simulink model "MBSE_PROJECT"  (R2020b)
settings: Solver=VariableStepAuto  StartTime=0.0  StopTime=10.0  RelTol=1e-3
undefined symbols (not defined in the file): sigbuilder_block
libraries: simulink x18
(part 1 of 2)
settings Model: Creator=99003757  LastModifiedBy=99003732

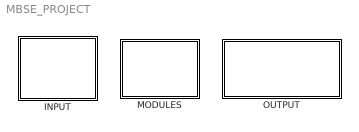
== system MBSE_PROJECT ==
  INPUT : Subsystem
  MODULES : Subsystem
  OUTPUT : Subsystem

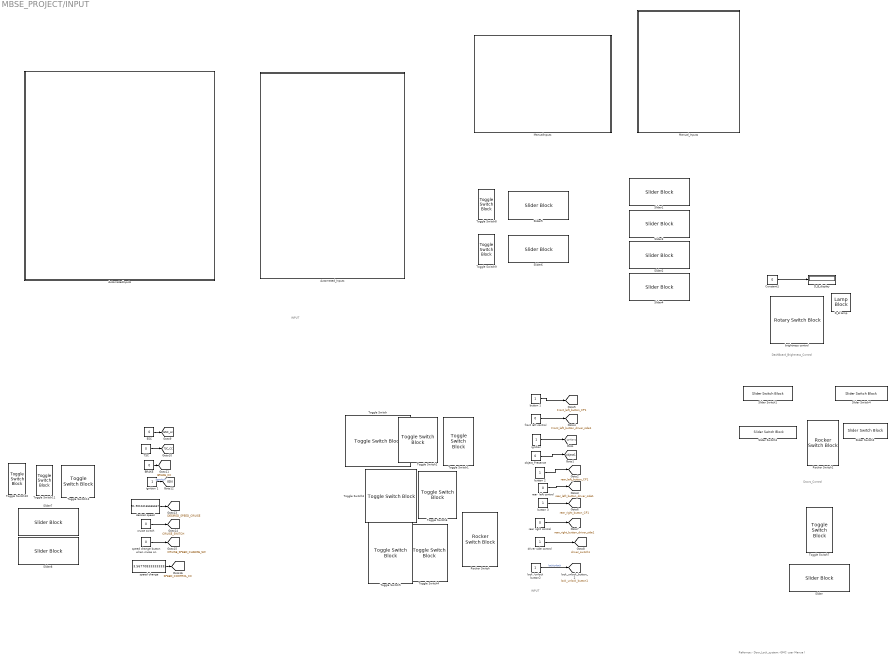
== system MBSE_PROJECT/INPUT ==
  note: INPUT
  note: INPUT
  note: DashBoard_Brightness_Control
  note: Doors_Control
  note: Refernce:-
      | Door_Lock_system:-GMC user Manua l
  AutomatedInputs : Subsystem
  Automated_Inputs : Subsystem
  BRAKE : Constant  Value=0
  Constant1 : Constant  Value=0
  D_B lamp : LampBlock
  D_B_display : Display
  ESC : Constant  Value=0
  ManualInputs : Subsystem
  Manual_Inputs : Subsystem
  Rocker Switch : RockerSwitchBlock  LabelPosition=Bottom
      settings: Values={{'Off', 'On'}, [0 1]}
  Rocker Switch1 : RockerSwitchBlock
      settings: Values={{'Off', 'On'}, [1 0]}
  Slider{,1..8} (9 alike) : SliderBlock
  Slider Switch{1..4} (4 alike) : SliderSwitchBlock
      settings: Values={{'unlock', 'lock'}, [0 1]}
  TSC : Constant  Value=0
  Toggle Switch{,1..12} (13 alike) : ToggleSwitchBlock
  brightness control : RotarySwitchBlock
      settings: Values={{'Off', 'very Low', 'Low', 'medium', 'high', 'very high'}, [0 1 2 3 4 5]}
  "button 1 " : Constant
  button 2 : Constant
  button 3 : Constant
  cruise switch : Constant  Value=0
  desired speed : Constant  Value=51.90104166666667
  driver side control : Constant
  front left control : Constant  Value=0
  "ignition " : Constant
  ignition 1 : Constant
  lock /unlock button2 : Constant
  object_Presence : Constant  Value=0
  rear  left control : Constant  Value=0
  rear right control : Constant  Value=0
  speed change : Constant  Value=3.567708333333333
  "speed change button when cruise on " : Constant  Value=0
  tag scope: BRAKE_CC=global, CRUISE_SPEED_CHANGE_SW=global, CRUISE_SWITCH=global, DESIRED_SPEED_CRUISE=global, ESC_cc=global, Front_left_button_CP1=global, Front_left_button_driver_side1=global, IGN=global, SPEED_CONTROL_CC=global, TSC_CC=global, driver_switch1=global, ignition1=global, lock_unlock_button1=global, object1=global, rear_left_button_CP1=global, rear_left_button_driver_side1=global, rear_right_button_CP1=global, rear_right_button_driver_side1=global
  wires:
  object_Presence/1 -> [object1]
  driver side control/1 -> [driver_switch1]
  Constant1/1 -> D_B_display/1
  button 3/1 -> [rear_right_button_CP1]
  rear right control/1 -> [rear_right_button_driver_side1]
  "ignition "/1 -> [ignition1]
  rear  left control/1 -> [rear_left_button_driver_side1]
  lock /unlock button2/1 -> [lock_unlock_button1]  "lock/unlock"
  button 2/1 -> [rear_left_button_CP1]
  front left control/1 -> [Front_left_button_driver_side1]
  "button 1 "/1 -> [Front_left_button_CP1]
  speed change/1 -> [SPEED_CONTROL_CC]
  desired speed/1 -> [DESIRED_SPEED_CRUISE]
  ESC/1 -> [ESC_cc]
  ignition 1/1 -> [IGN]  "igswitch"
  "speed change button when cruise on "/1 -> [CRUISE_SPEED_CHANGE_SW]
  BRAKE/1 -> [BRAKE_CC]
  TSC/1 -> [TSC_CC]
  cruise switch/1 -> [CRUISE_SWITCH]

== system MBSE_PROJECT/MODULES ==
  "\tPOWER_WINDOW" : Subsystem
  AirBagSystem : Subsystem
  CRUISE_CONTROL : Subsystem
  SeatRestraintSystem : Subsystem
  Subsystem2 : Subsystem
  Subsystem4 : Subsystem
  Tire Pressure Monitoring System : Subsystem

== system MBSE_PROJECT/OUTPUT ==
  note: Roof light
  note: Signal status
  note: roof light
  Cruise_output : Subsystem
  Lamp : LampBlock
  OUTPUT : Subsystem
  OUTPUT1 : Subsystem
  Outputs : Subsystem
  Outputs_Display : Subsystem
  TP1_Indicator : LampBlock
  TP2_Indicator : LampBlock
  TP3_Indicator : LampBlock
  TP4_Indicator : LampBlock
  automatic door lamp status : LampBlock
  delay lamp status : LampBlock

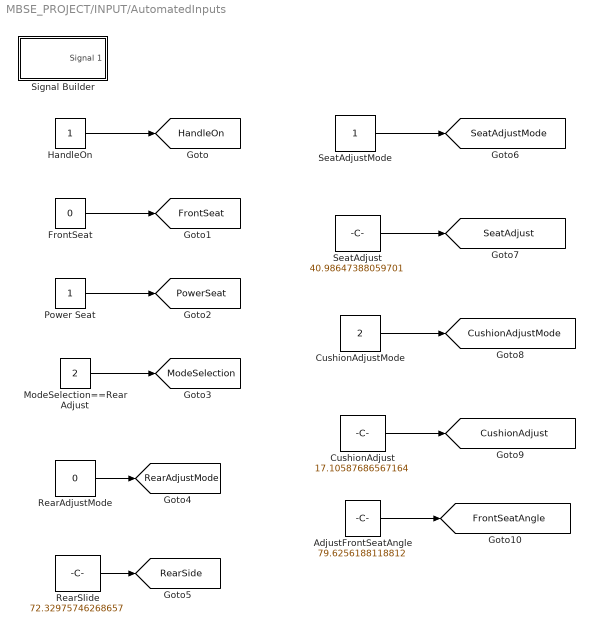
== system MBSE_PROJECT/INPUT/AutomatedInputs ==
  AdjustFrontSeatAngle : Constant  Value=79.6256188118812
  CushionAdjust : Constant  Value=17.10587686567164
  CushionAdjustMode : Constant  Value=2
  FrontSeat : Constant  Value=0
  HandleOn : Constant
  ModeSelection==RearAdjust : Constant  Value=2
  Power Seat : Constant
  RearAdjustMode : Constant  Value=0
  RearSlide : Constant  Value=72.32975746268657
  SeatAdjust : Constant  Value=40.98647388059701
  SeatAdjustMode : Constant
  Signal Builder : Subsystem  Tag=STV Subsys  LoadFcn=sigbuilder_block('load');  StartFcn=sigbuilder_block('start');  StopFcn=sigbuilder_block('stop');  ClipboardFcn=sigbuilder_block('clipboard');  mask(Sigbuilder block){tuvar=[0:10]}
      mask help: Simulink:masks:SigbuilderBlock_MD
      mask init:
      | if ~strcmp(get_param(bdroot(gcbh),'SimulationStatus'),'stopped') tuvar = sigbuilder_block('maskInit'); end
      settings: CopyFcn=sigbuilder_block('copy');  DeleteFcn=sigbuilder_block('delete');  ModelCloseFcn=sigbuilder_block('modelClose');  PreSaveFcn=sigbuilder_block('preSave');  PauseFcn=sigbuilder_block('pause');  ContinueFcn=sigbuilder_block('continue');  NameChangeFcn=sigbuilder_block('namechange');  OpenFcn=sigbuilder_block('open',[437.6 199.2 550.4 400 ]);  CloseFcn=sigbuilder_block('close');
      mask Display: plot(0, 0, 100, 100,[2, 2, 32, 32, 2], [68, 8, 8, 68, 68],[32, 2], [38, 38], [32, 19, 2],[53, 60, 44], [32, 17, 17, 2],[16, 16, 31, 31]);txt = getActiveGroup(gcbh);text(2, 100, txt,'verticalAlignment', 'top');
  tag scope: CushionAdjust=global, CushionAdjustMode=global, FrontSeat=global, FrontSeatAngle=global, HandleOn=global, ModeSelection=global, PowerSeat=global, RearAdjustMode=global, RearSide=global, SeatAdjust=global, SeatAdjustMode=global
  wires:
  HandleOn/1 -> [HandleOn]
  FrontSeat/1 -> [FrontSeat]
  Power Seat/1 -> [PowerSeat]
  ModeSelection==RearAdjust/1 -> [ModeSelection]
  RearAdjustMode/1 -> [RearAdjustMode]
  RearSlide/1 -> [RearSide]
  SeatAdjustMode/1 -> [SeatAdjustMode]
  SeatAdjust/1 -> [SeatAdjust]
  CushionAdjustMode/1 -> [CushionAdjustMode]
  CushionAdjust/1 -> [CushionAdjust]
  AdjustFrontSeatAngle/1 -> [FrontSeatAngle]

== system MBSE_PROJECT/INPUT/Automated_Inputs ==
  Driver : Constant
  L_Front : Constant
  L_Rear : Constant
  R_Rear : Constant  Value=0
  VehicleSpeed : Constant  Value=180
  YawRate : Constant  Value=100
  tag scope: Driver=global, L_Front=global, L_Rear=global, R_Rear=global, VehicleSpeed=global, YawRate=global
  wires:
  VehicleSpeed/1 -> [VehicleSpeed]
  YawRate/1 -> [YawRate]
  Driver/1 -> [Driver]
  L_Front/1 -> [L_Front]
  L_Rear/1 -> [L_Rear]
  R_Rear/1 -> [R_Rear]

== system MBSE_PROJECT/INPUT/ManualInputs ==
  Rotary Switch : RotarySwitchBlock  Commented=on
      settings: Values={{'RearAdjust', 'SeatAdjust', 'CushionAdjust', 'Lock'}, [0 1 2 3]}
  Slider to set the position of Frontseat : SliderBlock  Commented=on
  SliderForCushionAdjust : SliderBlock  Commented=on
  SliderForRearAdjust : SliderBlock  Commented=on
  SliderForSeatAdjust1 : SliderBlock  Commented=on
  Toggle Switch1 : ToggleSwitchBlock  Commented=on
      settings: Values={{'Off', 'On'}, [0 1]}
  Toggle Switch2 : ToggleSwitchBlock  Commented=on
      settings: Values={{'Off', 'On'}, [0 1]}
  Toggle Switch3 : ToggleSwitchBlock  Commented=on
      settings: Values={{'Off', 'On'}, [0 1]}

== system MBSE_PROJECT/INPUT/Manual_Inputs ==
  Vehicle_Speed : RotarySwitchBlock  Commented=on
      settings: Values={{'50kmph', '80kmph', '100kmph', '140kmph', '180kmph', '230kmph'}, [50 80 100 140 180 230]}
  YawRateMeasure : RotarySwitchBlock  Commented=on
      settings: Values={{'Forward', 'Turning'}, [50 100]}

== system MBSE_PROJECT/MODULES/	POWER_WINDOW ==
  Subsystem4 : Subsystem
  tag scope: FL_out=global, FL_warn=global, RL_out=global, RL_warn=global, RR_out=global, RR_warn=global, driver_side_output=global, driver_warn=global
  wires:
  Subsystem4/2(Out_FL) -> [FL_out]
  Subsystem4/1(Out_warn) -> [FL_warn]
  Subsystem4/4(Out_RL) -> [RL_out]
  Subsystem4/6(Out_RR) -> [RR_out]
  [object1] -> Subsystem4/2(object)
  [ignition1] -> Subsystem4/1(Ig_sw)
  Subsystem4/3(Out_RL_warn) -> [RL_warn]
  Subsystem4/8(Out_DC) -> [driver_side_output]
  Subsystem4/5(Out_RR_warn) -> [RR_warn]
  Subsystem4/7(Out_DC_warn) -> [driver_warn]

== system MBSE_PROJECT/MODULES/AirBagSystem ==
  AND : Logic  IconShape=distinctive  AllPortsSameDT=off  OutDataTypeStr=boolean
  AND1 : Logic  IconShape=distinctive  AllPortsSameDT=off  OutDataTypeStr=boolean
  ActivateAirBagSensor : MATLAB Function  TreatAsAtomicUnit=on
  DetectDeceleration : Subsystem
  FrontAirBagActivation : Subsystem  TreatAsAtomicUnit=on
  Side/Front : Subsystem
  SideAirBagActivation : Subsystem  TreatAsAtomicUnit=on
  wires:
  AND/1 -> FrontAirBagActivation/1(True), FrontAirBagActivation/Enable
  Side/Front/2(In_Front1) -> AND1/1
  ActivateAirBagSensor/1(AirBagSensor) -> AND1/2, AND/2
  Side/Front/1(In_Front) -> AND/1
  AND1/1 -> SideAirBagActivation/1(True), SideAirBagActivation/Enable
  DetectDeceleration/1(Out1) -> ActivateAirBagSensor/1(SuddenDeceleration)

== system MBSE_PROJECT/MODULES/CRUISE_CONTROL ==
  note: IGN
  Display : Display
  MATLAB Function : MATLAB Function  TreatAsAtomicUnit=on
  tag scope: output_cruise=global
  wires:
  [DESIRED_SPEED_CRUISE] -> MATLAB Function/5(DESIRED_SPEED_CRUISE)
  [BRAKE_CC] -> MATLAB Function/3(BRAKE_CC)
  [CRUISE_SWITCH] -> MATLAB Function/6(cs)
  [ESC_cc] -> MATLAB Function/1(ESC_CC)
  [SPEED_CONTROL_CC] -> MATLAB Function/8(speedch)
  MATLAB Function/1(y) -> [output_cruise], Display/1  "output"
  [TSC_CC] -> MATLAB Function/2(TSC_CC)
  [IGN] -> MATLAB Function/4(IGN)
  [CRUISE_SPEED_CHANGE_SW] -> MATLAB Function/7(CRUISE_SPEED_CHANGE_SW)

== system MBSE_PROJECT/MODULES/SeatRestraintSystem ==
  Front Seat : Subsystem  TreatAsAtomicUnit=on
  Handle/Power/Front : Subsystem
  PowerSeat : Subsystem
  wires:
  Handle/Power/Front/1(FrontEnable) -> Front Seat/Enable, Front Seat/1(ConditionCheck)
  Handle/Power/Front/2(PowerSeatEnable) -> PowerSeat/1(Enable)

== system MBSE_PROJECT/MODULES/Subsystem2 ==
  In1 : Inport
  CloseValue : Constant  Value=0
  OpenValue : Constant  Value=100
  Subsystem : Subsystem
  Subsystem1 : Subsystem
  enabling system : Subsystem
  tag scope: output1=global, output2=global
  wires:
  enabling system/1(Outport) -> Subsystem1/1(Enable)
  enabling system/2(enableO) -> Subsystem/1(Enable)
  CloseValue/1 -> Subsystem/2(Inport)
  OpenValue/1 -> Subsystem1/2(Inport)
  Subsystem/1(Outport) -> [output2]
  Subsystem1/1(Outport) -> [output1]

== system MBSE_PROJECT/MODULES/Subsystem4 ==
  AND : Logic  IconShape=distinctive  AllPortsSameDT=off  OutDataTypeStr=boolean
  AutomaticDoorLock : Subsystem
  Compare To Constant : simulink/Logic and Bit Operations/Compare To Constant  relop=>  const=0  OutDataTypeStr=boolean
  Display : Display
  Display1 : Display
  OR1 : Logic  Operator=OR  IconShape=distinctive  AllPortsSameDT=off  OutDataTypeStr=boolean
  delay system door lock and interior light subsystem : Subsystem
  wires:
  AutomaticDoorLock/1(Out1) -> AND/1
  AND/1 -> OR1/1, Display/1
  AutomaticDoorLock/2(Out2) -> AND/2
  Compare To Constant/1 -> OR1/2
  OR1/1 -> Display1/1
  delay system door lock and interior light subsystem/1(Out1) -> Compare To Constant/1

== system MBSE_PROJECT/MODULES/Tire Pressure Monitoring System ==
  TP_Monitoring : Subsystem
  Tier1State : Display
  Tier2State : Display
  Tier3State : Display
  Tier4State : Display
  tierPressure1 : Constant  Value=87.46448863636364
  tierPressure2 : Constant  Value=75.64630681818181
  tierPressure3 : Constant  Value=78.37357954545455
  tierPressure4 : Constant  Value=86.10085227272727
  wires:
  TP_Monitoring/2(Out2) -> Tier2State/1
  tierPressure4/1 -> TP_Monitoring/4(tierPressure4a), TP_Monitoring/8(tierPressure4b)
  TP_Monitoring/1(Out1) -> Tier1State/1
  tierPressure1/1 -> TP_Monitoring/5(tierPressure1b), TP_Monitoring/1(tierPressure1a)
  tierPressure3/1 -> TP_Monitoring/3(tierPressure3a), TP_Monitoring/7(tierPressure3b)
  TP_Monitoring/3(Out3) -> Tier3State/1
  tierPressure2/1 -> TP_Monitoring/6(tierPressure2b), TP_Monitoring/2(tierPressure2a)
  TP_Monitoring/4(Out4) -> Tier4State/1

== system MBSE_PROJECT/OUTPUT/Cruise_output ==
  Gauge : CircularGaugeBlock
  Scope : Scope
  wires:
  [output_cruise] -> Scope/1

== system MBSE_PROJECT/OUTPUT/OUTPUT ==
  Output_window_scope : Scope  NumInputPorts=4
  Warning_Scope : Scope  NumInputPorts=4
  wires:
  [RR_warn] -> Warning_Scope/3
  [RL_warn] -> Warning_Scope/2
  [FL_warn] -> Warning_Scope/1
  [FL_out] -> Output_window_scope/1
  [RL_out] -> Output_window_scope/2
  [RR_out] -> Output_window_scope/3
  [driver_side_output] -> Output_window_scope/4
  [driver_warn] -> Warning_Scope/4

== system MBSE_PROJECT/OUTPUT/OUTPUT1 ==
  Display : Display
  Display1 : Display
  wires:
  [output2] -> Display1/1
  [output1] -> Display/1

== system MBSE_PROJECT/OUTPUT/Outputs ==
  CushionAdjust2 : LampBlock
  CushionAngle : Display
  Front Seat Adjust : LampBlock
  FrontAngle : Display
  RearAdjust : LampBlock
  RearAngle : Display
  SeatAdjust1 : LampBlock
  SeatAngle : Display
  wires:
  [CushionAngle] -> CushionAngle/1
  [SeatAngle] -> SeatAngle/1
  [RearAngle] -> RearAngle/1
  [FrontAngle] -> FrontAngle/1

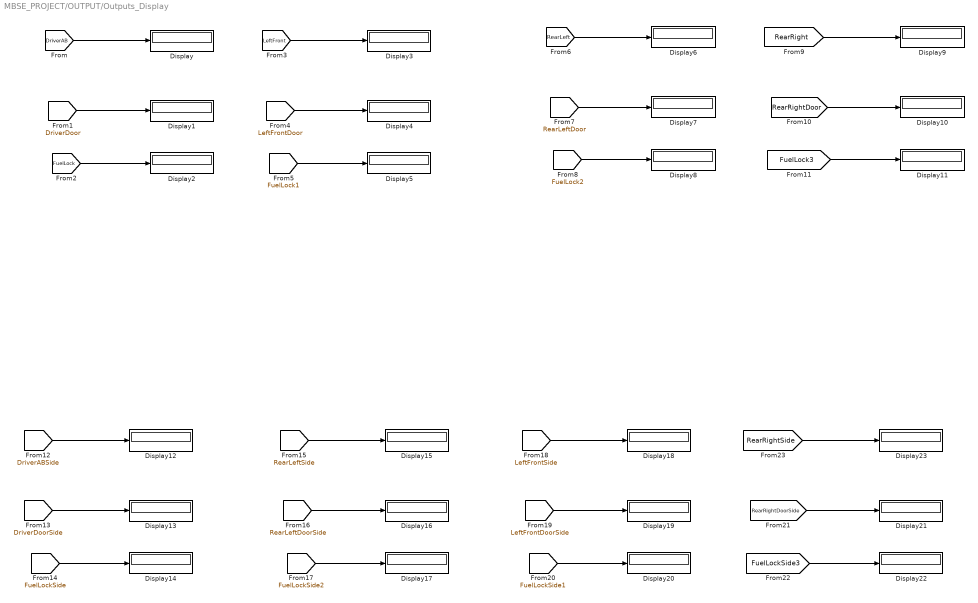
== system MBSE_PROJECT/OUTPUT/Outputs_Display ==
  Display{,1..23} (24 alike) : Display
  wires:
  [DriverDoor] -> Display1/1
  [FuelLock] -> Display2/1
  [DriverAB] -> Display/1
  [FuelLock1] -> Display5/1
  [LeftFront] -> Display3/1
  [LeftFrontDoor] -> Display4/1
  [RearLeft] -> Display6/1
  [RearLeftDoor] -> Display7/1
  [FuelLock2] -> Display8/1
  [RearRightDoor] -> Display10/1
  [FuelLock3] -> Display11/1
  [RearRight] -> Display9/1
  [FuelLockSide] -> Display14/1
  [DriverABSide] -> Display12/1
  [DriverDoorSide] -> Display13/1
  [RearLeftDoorSide] -> Display16/1
  [FuelLockSide2] -> Display17/1
  [RearLeftSide] -> Display15/1
  [LeftFrontSide] -> Display18/1
  [LeftFrontDoorSide] -> Display19/1
  [FuelLockSide1] -> Display20/1
  [RearRightSide] -> Display23/1
  [RearRightDoorSide] -> Display21/1
  [FuelLockSide3] -> Display22/1

== system MBSE_PROJECT/INPUT/AutomatedInputs/Signal Builder ==
  Demux : Demux  Tag=STV Demux  Outputs=1
      settings: DisplayOption=none
  FromWs : FromWorkspace  Tag=STV FromWs  VariableName=tuvar
      SigBuilderData=|
      | common.afterFinalStr = 'Extrapolate'
      | common.sampleTime = 0
      | dataSet.timeRange = [0 10]
      | dataSet.name = 'Group 1'
      | sbobj.Groups.Name = 'Group 1'
      | sbobj.Groups.Signals.Name = 'Signal 1'
      | sbobj.Groups.Signals.XData = [0 4 4 6 6 10]
      | sbobj.Groups.Signals.YData = [0 0 1 1 0 0]
  Signal 1 : Outport  Tag=STV Outport
  wires:
  Demux/1 -> Signal 1/1
  FromWs/1 -> Demux/1

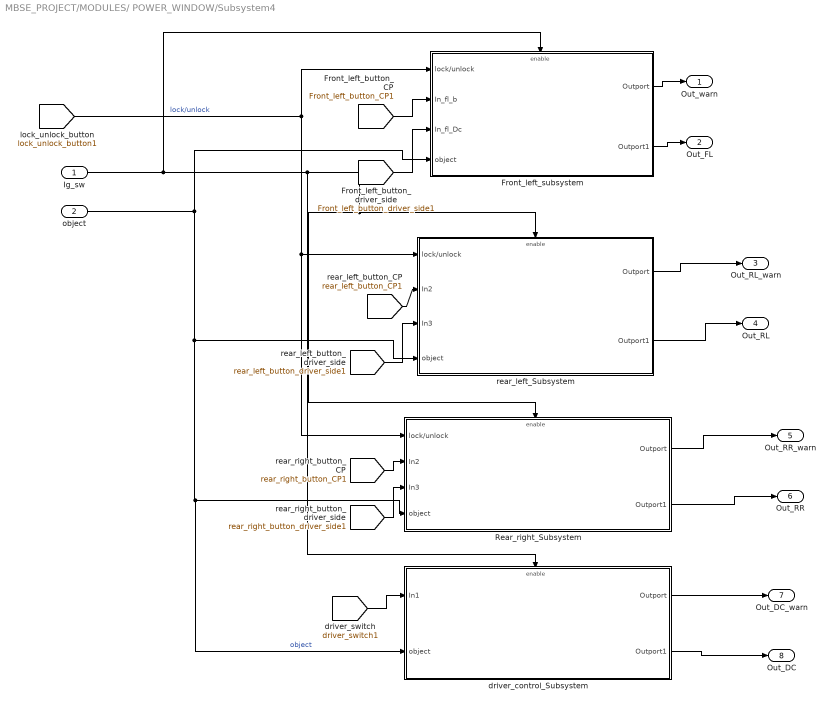
== system MBSE_PROJECT/MODULES/	POWER_WINDOW/Subsystem4 ==
  Ig_sw : Inport
  object : Inport  Port=2
  Front_left_subsystem : Subsystem
  Rear_right_Subsystem : Subsystem
  driver_control_Subsystem : Subsystem
  rear_left_Subsystem : Subsystem
  Out_warn : Outport
  Out_FL : Outport  Port=2
  Out_RL_warn : Outport  Port=3
  Out_RL : Outport  Port=4
  Out_RR_warn : Outport  Port=5
  Out_RR : Outport  Port=6
  Out_DC_warn : Outport  Port=7
  Out_DC : Outport  Port=8
  wires:
  [lock_unlock_button1] -> Front_left_subsystem/1(lock/unlock), Rear_right_Subsystem/1(lock/unlock), rear_left_Subsystem/1(lock/unlock)  "lock/unlock"
  Ig_sw/1 -> Rear_right_Subsystem/Enable, rear_left_Subsystem/Enable, driver_control_Subsystem/Enable, Front_left_subsystem/Enable
  object/1 -> Front_left_subsystem/4(object), driver_control_Subsystem/2(object), Rear_right_Subsystem/4(object), rear_left_Subsystem/4(object)  "object"
  Front_left_subsystem/2(Outport1) -> Out_FL/1
  Front_left_subsystem/1(Outport) -> Out_warn/1
  rear_left_Subsystem/2(Outport1) -> Out_RL/1
  rear_left_Subsystem/1(Outport) -> Out_RL_warn/1
  Rear_right_Subsystem/2(Outport1) -> Out_RR/1
  Rear_right_Subsystem/1(Outport) -> Out_RR_warn/1
  driver_control_Subsystem/2(Outport1) -> Out_DC/1
  driver_control_Subsystem/1(Outport) -> Out_DC_warn/1
  [Front_left_button_CP1] -> Front_left_subsystem/2(In_fl_b)
  [Front_left_button_driver_side1] -> Front_left_subsystem/3(In_fl_Dc)
  [rear_left_button_CP1] -> rear_left_Subsystem/2(In2)
  [rear_left_button_driver_side1] -> rear_left_Subsystem/3(In3)
  [rear_right_button_CP1] -> Rear_right_Subsystem/2(In2)
  [rear_right_button_driver_side1] -> Rear_right_Subsystem/3(In3)
  [driver_switch1] -> driver_control_Subsystem/1(In1)

== system MBSE_PROJECT/MODULES/AirBagSystem/DetectDeceleration ==
  ConstantVehicleSpeed : Constant  Value=50
  DetectDeceleration : Sum  Inputs=+-
  SuddenDeceleration : RelationalOperator  OutDataTypeStr=boolean  RndMeth=Simplest
  Value : Constant  Value=60
  Out1 : Outport
  wires:
  DetectDeceleration/1 -> SuddenDeceleration/1
  Value/1 -> SuddenDeceleration/2
  SuddenDeceleration/1 -> Out1/1
  [VehicleSpeed] -> DetectDeceleration/1
  ConstantVehicleSpeed/1 -> DetectDeceleration/2

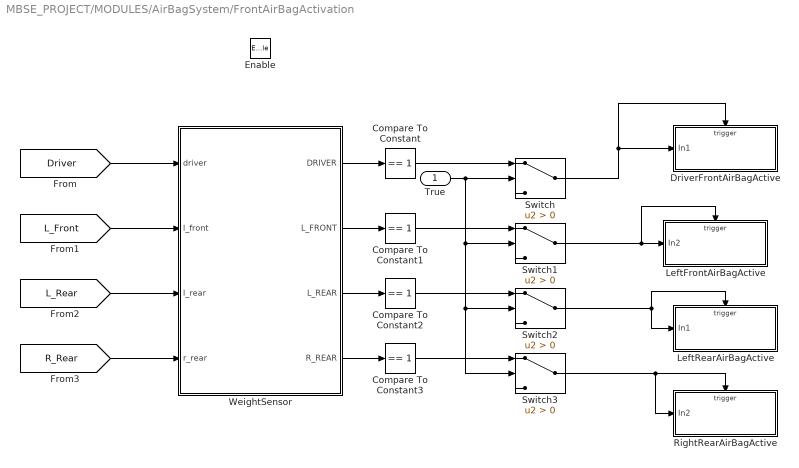
== system MBSE_PROJECT/MODULES/AirBagSystem/FrontAirBagActivation ==
  True : Inport
  Enable : EnablePort
  Compare To Constant{,1..3} (4 alike) : simulink/Logic and Bit Operations/Compare To Constant  relop===  const=1  OutDataTypeStr=boolean
  DriverFrontAirBagActive : Subsystem  TreatAsAtomicUnit=on
  LeftFrontAirBagActive : Subsystem  TreatAsAtomicUnit=on
  LeftRearAirBagActive : Subsystem  TreatAsAtomicUnit=on
  RightRearAirBagActive : Subsystem  TreatAsAtomicUnit=on
  Switch{,1..3} (4 alike) : Switch  Criteria=u2 > Threshold
  WeightSensor : MATLAB Function  TreatAsAtomicUnit=on
  wires:
  WeightSensor/2(L_FRONT) -> Compare To Constant1/1
  [L_Front] -> WeightSensor/2(l_front)
  [Driver] -> WeightSensor/1(driver)
  WeightSensor/1(DRIVER) -> Compare To Constant/1
  WeightSensor/3(L_REAR) -> Compare To Constant2/1
  WeightSensor/4(R_REAR) -> Compare To Constant3/1
  [R_Rear] -> WeightSensor/4(r_rear)
  [L_Rear] -> WeightSensor/3(l_rear)
  True/1 -> Switch3/2, Switch2/2, Switch1/2, Switch/2
  Compare To Constant/1 -> Switch/1
  Switch/1 -> DriverFrontAirBagActive/Trigger, DriverFrontAirBagActive/1(In1)
  Compare To Constant1/1 -> Switch1/1
  Switch1/1 -> LeftFrontAirBagActive/1(In2), LeftFrontAirBagActive/Trigger
  Compare To Constant2/1 -> Switch2/1
  Switch2/1 -> LeftRearAirBagActive/Trigger, LeftRearAirBagActive/1(In1)
  Compare To Constant3/1 -> Switch3/1
  Switch3/1 -> RightRearAirBagActive/1(In2), RightRearAirBagActive/Trigger

== system MBSE_PROJECT/MODULES/AirBagSystem/Side//Front ==
  CheckYawRateForFront : RelationalOperator  Operator===  OutDataTypeStr=boolean  RndMeth=Simplest
  CheckYawRateForSide : RelationalOperator  Operator===  OutDataTypeStr=boolean  RndMeth=Simplest
  Val_Front : Constant  Value=50
  Val_Side : Constant  Value=100
  In_Front : Outport
  In_Front1 : Outport  Port=2
  wires:
  Val_Front/1 -> CheckYawRateForFront/2
  [YawRate] -> CheckYawRateForSide/1, CheckYawRateForFront/1
  CheckYawRateForFront/1 -> In_Front/1
  Val_Side/1 -> CheckYawRateForSide/2
  CheckYawRateForSide/1 -> In_Front1/1

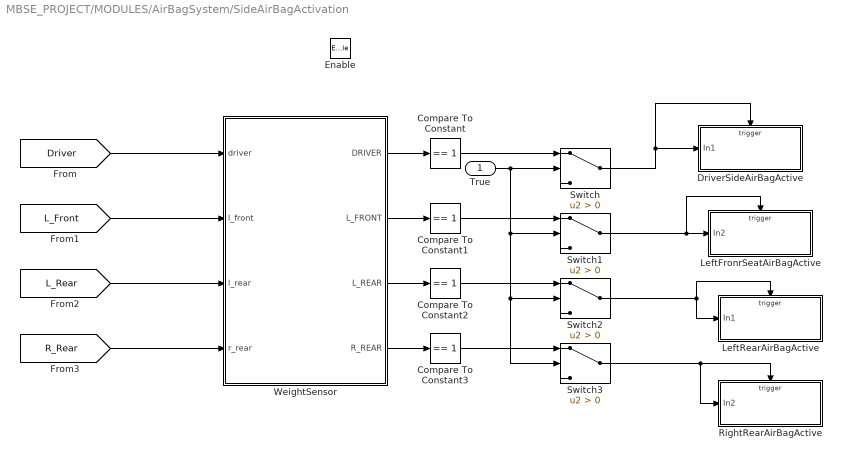
== system MBSE_PROJECT/MODULES/AirBagSystem/SideAirBagActivation ==
  True : Inport
  Enable : EnablePort
  Compare To Constant{,1..3} (4 alike) : simulink/Logic and Bit Operations/Compare To Constant  relop===  const=1  OutDataTypeStr=boolean
  DriverSideAirBagActive : Subsystem  TreatAsAtomicUnit=on
  LeftFronrSeatAirBagActive : Subsystem  TreatAsAtomicUnit=on
  LeftRearAirBagActive : Subsystem  TreatAsAtomicUnit=on
  RightRearAirBagActive : Subsystem  TreatAsAtomicUnit=on
  Switch{,1..3} (4 alike) : Switch  Criteria=u2 > Threshold
  WeightSensor : MATLAB Function  TreatAsAtomicUnit=on
  wires:
  Switch2/1 -> LeftRearAirBagActive/Trigger, LeftRearAirBagActive/1(In1)
  WeightSensor/2(L_FRONT) -> Compare To Constant1/1
  WeightSensor/3(L_REAR) -> Compare To Constant2/1
  WeightSensor/4(R_REAR) -> Compare To Constant3/1
  [L_Front] -> WeightSensor/2(l_front)
  Compare To Constant1/1 -> Switch1/1
  [R_Rear] -> WeightSensor/4(r_rear)
  True/1 -> Switch3/2, Switch2/2, Switch1/2, Switch/2
  Switch/1 -> DriverSideAirBagActive/Trigger, DriverSideAirBagActive/1(In1)
  [Driver] -> WeightSensor/1(driver)
  Switch1/1 -> LeftFronrSeatAirBagActive/1(In2), LeftFronrSeatAirBagActive/Trigger
  [L_Rear] -> WeightSensor/3(l_rear)
  WeightSensor/1(DRIVER) -> Compare To Constant/1
  Compare To Constant3/1 -> Switch3/1
  Compare To Constant2/1 -> Switch2/1
  Compare To Constant/1 -> Switch/1
  Switch3/1 -> RightRearAirBagActive/1(In2), RightRearAirBagActive/Trigger

== system MBSE_PROJECT/MODULES/SeatRestraintSystem/Front Seat ==
  ConditionCheck : Inport
  Enable : EnablePort
  Enable Adjustment mode1 : Switch  Criteria=u2 > Threshold
  FrontSeatAdjusted : simulink/Logic and Bit Operations/Compare To Constant  relop=>  const=0  OutDataTypeStr=boolean
  tag scope: FrontAngle=global
  wires:
  [FrontSeatAngle] -> Enable Adjustment mode1/1
  ConditionCheck/1 -> Enable Adjustment mode1/2
  Enable Adjustment mode1/1 -> FrontSeatAdjusted/1
  FrontSeatAdjusted/1 -> [FrontAngle]

== system MBSE_PROJECT/MODULES/SeatRestraintSystem/Handle//Power//Front ==
  AND : Logic  IconShape=distinctive  AllPortsSameDT=off  OutDataTypeStr=boolean
  AND1 : Logic  IconShape=distinctive  AllPortsSameDT=off  OutDataTypeStr=boolean
  FrontEnable : Outport
  PowerSeatEnable : Outport  Port=2
  wires:
  AND/1 -> FrontEnable/1
  [PowerSeat] -> AND1/2
  [HandleOn] -> AND1/1, AND/1
  [FrontSeat] -> AND/2
  AND1/1 -> PowerSeatEnable/1

== system MBSE_PROJECT/MODULES/SeatRestraintSystem/PowerSeat ==
  Enable : Inport
  PowerSeat : Subsystem  TreatAsAtomicUnit=on
  wires:
  Enable/1 -> PowerSeat/Enable, PowerSeat/1(ConditionCheck2), PowerSeat/2(ConditionCheck3), PowerSeat/3(RearAdjEnable), PowerSeat/5(CushionAdjEnable), PowerSeat/4(SeatAdjEnable)

== system MBSE_PROJECT/MODULES/Subsystem2/Subsystem ==
  Enable : Inport
  Inport : Inport  Port=2
  Enabled Subsystem : Subsystem  TreatAsAtomicUnit=on
  Outport : Outport
  wires:
  Enabled Subsystem/1(Outport) -> Outport/1
  Inport/1 -> Enabled Subsystem/1(In1)
  Enable/1 -> Enabled Subsystem/Enable

== system MBSE_PROJECT/MODULES/Subsystem2/Subsystem1 ==
  Enable : Inport
  Inport : Inport  Port=2
  Enabled Subsystem1 : Subsystem  TreatAsAtomicUnit=on
  Outport : Outport
  wires:
  Inport/1 -> Enabled Subsystem1/1(In1)
  Enabled Subsystem1/1(Outport) -> Outport/1
  Enable/1 -> Enabled Subsystem1/Enable

== system MBSE_PROJECT/MODULES/Subsystem2/enabling system ==
  Chart : Stateflow chart  TreatAsAtomicUnit=on
      settings: PortSchema="{\"entries\":[{\"content\":{\"sides\":[{\"content\":{\"connectorIds\":[\"In2\",\"In1\"]},\"type\":\"ConnectorPlacement.EquallySpacedRectSide\",\"uuid\":\"e77fb548-5411-4dff-a09c-dcff2e4e83fa\"},{\"content\":{\"connectorIds\":[\"Out1\",\"Out2\"],\"side\":\"RIGHT\"},\"type\":\"ConnectorPlacement.EquallySpacedRectSide\",\"uuid\":\"fb2d12f5-730f-4265-a3f8-30409b75040e\"},{\"content\":{\"connectorIds\":[],\"side\":\"TOP\"},\"type\":\"ConnectorPlacement.EquallySpacedRectSide\",\"uuid\":\"5ec706c6-4a0b-4294-a183-09121d2d4adc\"},{\"content\":{\"connectorIds\":[],\"side\":\"HIDDEN\"},\"type\":\"ConnectorPlacement.EquallySpacedRectSide\",\"uuid\":\"e64ccab7-f9d3-41b0-81fa-c7461dca4746\"}]},\"type\":\"ConnectorPlacement.EquallySpacedConnector\",\"uuid\":\"e8c87857-404b-4a97-9417-fff31936aad1\"}],\"packageUris\":[\"http://schema.mathworks.com/mf0/Connector/R2020b\"],\"version\":\"1.0\"}"
  Close : Constant
  Open : Constant  Value=0
  Outport : Outport
  enableO : Outport  Port=2
  wires:
  Chart/1(enableC) -> Outport/1
  Close/1 -> Chart/1(closeButton)
  Chart/2(enableO) -> enableO/1
  Open/1 -> Chart/2(openButton)

== system MBSE_PROJECT/MODULES/Subsystem4/AutomaticDoorLock ==
  A_D_accln : Constant  Value=15.43496621621622
  A_D_ignition : Constant
  Constant : Constant
  If : If  IfExpression=u1>=13  ElseIfExpressions=u1<13  ShowElse=off
  If Action Subsystem : Subsystem  TreatAsAtomicUnit=on
  If Action Subsystem1 : Subsystem  TreatAsAtomicUnit=on
  OR : Logic  Operator=OR  IconShape=distinctive  AllPortsSameDT=off  OutDataTypeStr=boolean
  reset : Constant  Value=0
  Out1 : Outport
  Out2 : Outport  Port=2
  wires:
  Constant/1 -> If Action Subsystem/1(In1)
  If Action Subsystem/1(Out1) -> OR/1
  If/1 -> If Action Subsystem/Action
  If/2 -> If Action Subsystem1/Action
  If Action Subsystem1/1(Out1) -> OR/2
  A_D_ignition/1 -> Out1/1
  OR/1 -> Out2/1
  A_D_accln/1 -> If/1
  reset/1 -> If Action Subsystem1/1(In1)

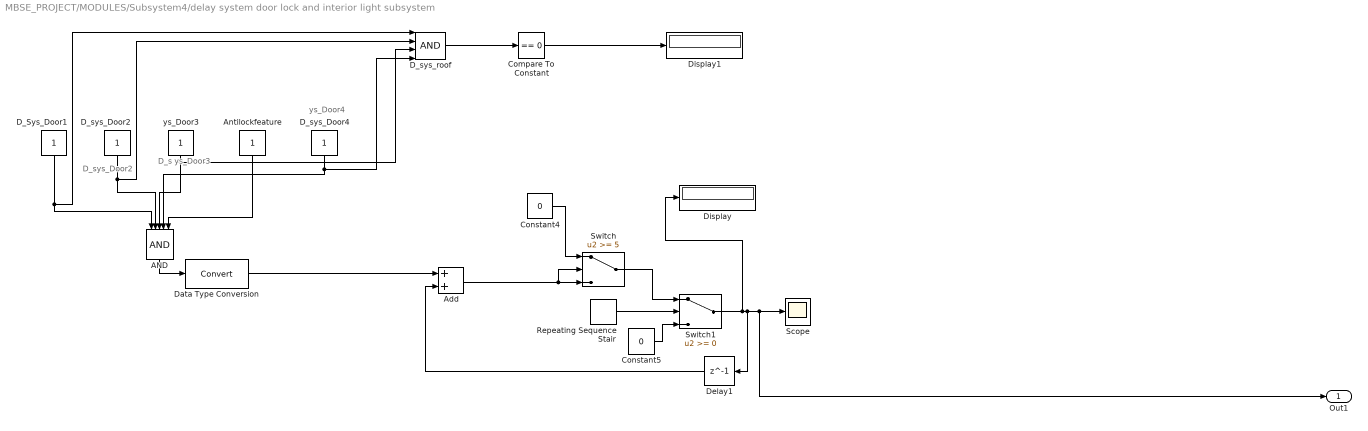
== system MBSE_PROJECT/MODULES/Subsystem4/delay system door lock and interior light subsystem ==
  note: D_s ys_Door3
  note: D_sys_Door2
  note: ys_Door4
  AND : Logic  Inputs=5  IconShape=distinctive  AllPortsSameDT=off  OutDataTypeStr=boolean
  Add : Sum
  Antilockfeature : Constant
  Compare To Constant : simulink/Logic and Bit Operations/Compare To Constant  relop===  const=0  OutDataTypeStr=boolean
  Constant4 : Constant  Value=0
  Constant5 : Constant  Value=0
  D_Sys_Door1 : Constant
  D_sys_Door2 : Constant
  D_sys_Door4 : Constant
  D_sys_roof : Logic  Inputs=4  IconShape=distinctive  AllPortsSameDT=off  OutDataTypeStr=boolean
  Data Type Conversion : DataTypeConversion
  Delay1 : Delay  DelayLength=1
  Display : Display
  Display1 : Display
  Repeating Sequence Stair : simulink/Sources/Repeating Sequence Stair  OutValues=[1 1]  tsamp=-1  OutMin=[]  OutMax=[]  OutDataTypeStr=double  OutputDataTypeScalingMode=double  OutDataType=fixdt(0,8)  ConRadixGroup=Best Precision: Vector-wise  OutScaling=2^-12
  Scope : Scope
  Switch : Switch  Threshold=5
  Switch1 : Switch
  ys_Door3 : Constant
  Out1 : Outport
  wires:
  Switch1/1 -> Scope/1, Out1/1, Delay1/1, Display/1
  Antilockfeature/1 -> AND/5
  Repeating Sequence Stair/1 -> Switch1/2
  Delay1/1 -> Add/2
  Constant5/1 -> Switch1/3
  Constant4/1 -> Switch/1
  Add/1 -> Switch/2, Switch/3
  Switch/1 -> Switch1/1
  AND/1 -> Data Type Conversion/1
  ys_Door3/1 -> D_sys_roof/3, AND/3
  D_sys_Door4/1 -> D_sys_roof/4, AND/4
  D_sys_roof/1 -> Compare To Constant/1
  D_Sys_Door1/1 -> D_sys_roof/1, AND/1
  D_sys_Door2/1 -> D_sys_roof/2, AND/2
  Compare To Constant/1 -> Display1/1
  Data Type Conversion/1 -> Add/1

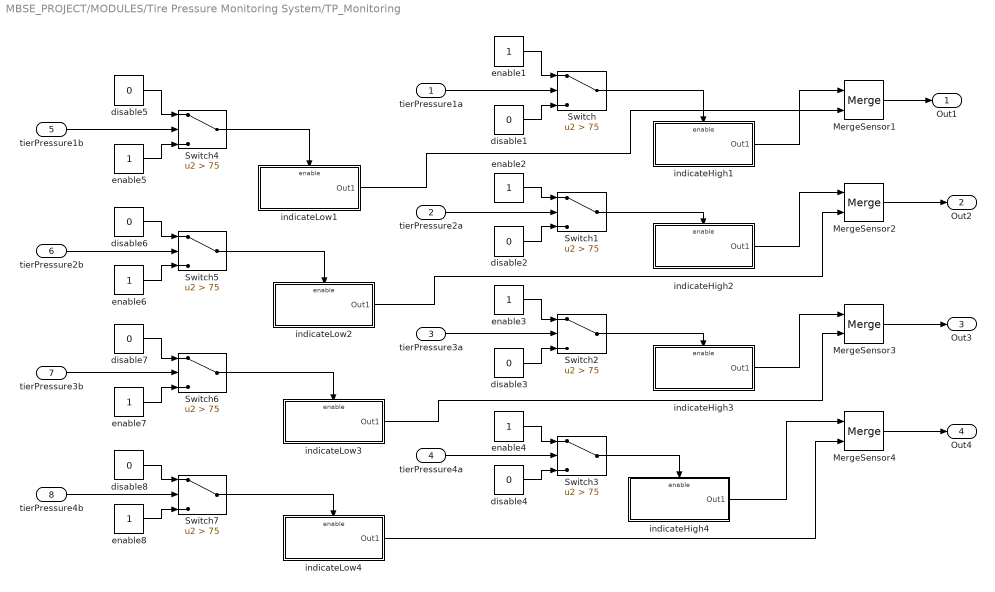
== system MBSE_PROJECT/MODULES/Tire Pressure Monitoring System/TP_Monitoring ==
  tierPressure1a : Inport
  tierPressure2a : Inport  Port=2
  tierPressure3a : Inport  Port=3
  tierPressure4a : Inport  Port=4
  tierPressure1b : Inport  Port=5
  tierPressure2b : Inport  Port=6
  tierPressure3b : Inport  Port=7
  tierPressure4b : Inport  Port=8
  MergeSensor{1..4} (4 alike) : Merge
  Switch{,1..7} (8 alike) : Switch  Criteria=u2 > Threshold  Threshold=75
  disable{1..8} (8 alike) : Constant  Value=0
  enable{1..8} (8 alike) : Constant
  indicateHigh1 : Subsystem  TreatAsAtomicUnit=on
  indicateHigh2 : Subsystem  TreatAsAtomicUnit=on
  indicateHigh3 : Subsystem  TreatAsAtomicUnit=on
  indicateHigh4 : Subsystem  TreatAsAtomicUnit=on
  indicateLow1 : Subsystem  TreatAsAtomicUnit=on
  indicateLow2 : Subsystem  TreatAsAtomicUnit=on
  indicateLow3 : Subsystem  TreatAsAtomicUnit=on
  indicateLow4 : Subsystem  TreatAsAtomicUnit=on
  Out1 : Outport
  Out2 : Outport  Port=2
  Out3 : Outport  Port=3
  Out4 : Outport  Port=4
  wires:
  enable1/1 -> Switch/1
  tierPressure3a/1 -> Switch2/2
  disable1/1 -> Switch/3
  disable3/1 -> Switch2/3
  enable2/1 -> Switch1/1
  tierPressure1a/1 -> Switch/2
  disable4/1 -> Switch3/3
  disable2/1 -> Switch1/3
  enable4/1 -> Switch3/1
  tierPressure2a/1 -> Switch1/2
  tierPressure4a/1 -> Switch3/2
  enable3/1 -> Switch2/1
  disable8/1 -> Switch7/1
  enable8/1 -> Switch7/3
  disable6/1 -> Switch5/1
  enable6/1 -> Switch5/3
  enable7/1 -> Switch6/3
  enable5/1 -> Switch4/3
  disable5/1 -> Switch4/1
  tierPressure2b/1 -> Switch5/2
  tierPressure3b/1 -> Switch6/2
  tierPressure1b/1 -> Switch4/2
  disable7/1 -> Switch6/1
  tierPressure4b/1 -> Switch7/2
  MergeSensor1/1 -> Out1/1
  MergeSensor2/1 -> Out2/1
  MergeSensor3/1 -> Out3/1
  MergeSensor4/1 -> Out4/1
  Switch3/1 -> indicateHigh4/Enable
  Switch2/1 -> indicateHigh3/Enable
  Switch1/1 -> indicateHigh2/Enable
  Switch/1 -> indicateHigh1/Enable
  Switch7/1 -> indicateLow4/Enable
  Switch6/1 -> indicateLow3/Enable
  Switch5/1 -> indicateLow2/Enable
  Switch4/1 -> indicateLow1/Enable
  indicateHigh1/1(Out1) -> MergeSensor1/1
  indicateLow1/1(Out1) -> MergeSensor1/2
  indicateHigh2/1(Out1) -> MergeSensor2/1
  indicateLow2/1(Out1) -> MergeSensor2/2
  indicateHigh3/1(Out1) -> MergeSensor3/1
  indicateLow3/1(Out1) -> MergeSensor3/2
  indicateHigh4/1(Out1) -> MergeSensor4/1
  indicateLow4/1(Out1) -> MergeSensor4/2

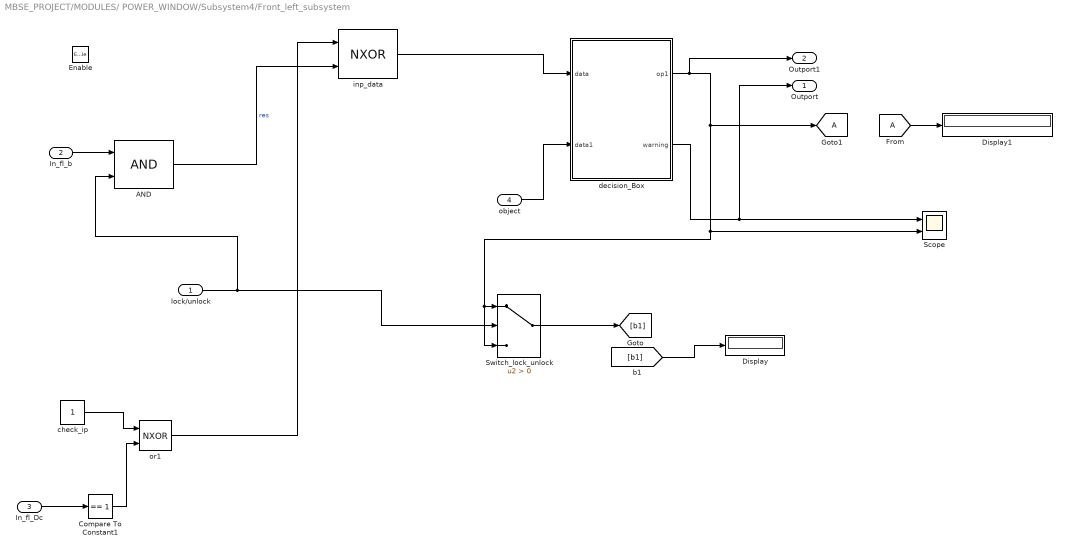
== system MBSE_PROJECT/MODULES/	POWER_WINDOW/Subsystem4/Front_left_subsystem ==
  lock/unlock : Inport
  In_fl_b : Inport  Port=2
  In_fl_Dc : Inport  Port=3
  object : Inport  Port=4
  Enable : EnablePort
  AND : Logic  IconShape=distinctive  AllPortsSameDT=off  OutDataTypeStr=boolean
  Compare To Constant1 : simulink/Logic and Bit Operations/Compare To Constant  relop===  const=1  OutDataTypeStr=boolean
  Display : Display
  Display1 : Display
  Scope : Scope  NumInputPorts=2
  Switch_lock_unlock : Switch  Criteria=u2 > Threshold
  check_ip : Constant
  decision_Box : Stateflow chart  TreatAsAtomicUnit=on
  inp_data : Logic  Operator=NXOR  IconShape=distinctive  AllPortsSameDT=off  OutDataTypeStr=boolean
  or1 : Logic  Operator=NXOR  IconShape=distinctive  AllPortsSameDT=off  OutDataTypeStr=boolean
  Outport : Outport
  Outport1 : Outport  Port=2
  tag scope: A=global
  wires:
  In_fl_b/1 -> AND/1
  check_ip/1 -> or1/1
  Switch_lock_unlock/1 -> [b1]
  Compare To Constant1/1 -> or1/2
  [b1] -> Display/1
  decision_Box/1(op1) -> Outport1/1, Switch_lock_unlock/3, Switch_lock_unlock/1, Scope/2, [A]
  decision_Box/2(warning) -> Outport/1, Scope/1
  object/1 -> decision_Box/2(data1)
  AND/1 -> inp_data/2  "res"
  or1/1 -> inp_data/1
  lock/unlock/1 -> AND/2, Switch_lock_unlock/2
  [A] -> Display1/1
  inp_data/1 -> decision_Box/1(data)
  In_fl_Dc/1 -> Compare To Constant1/1

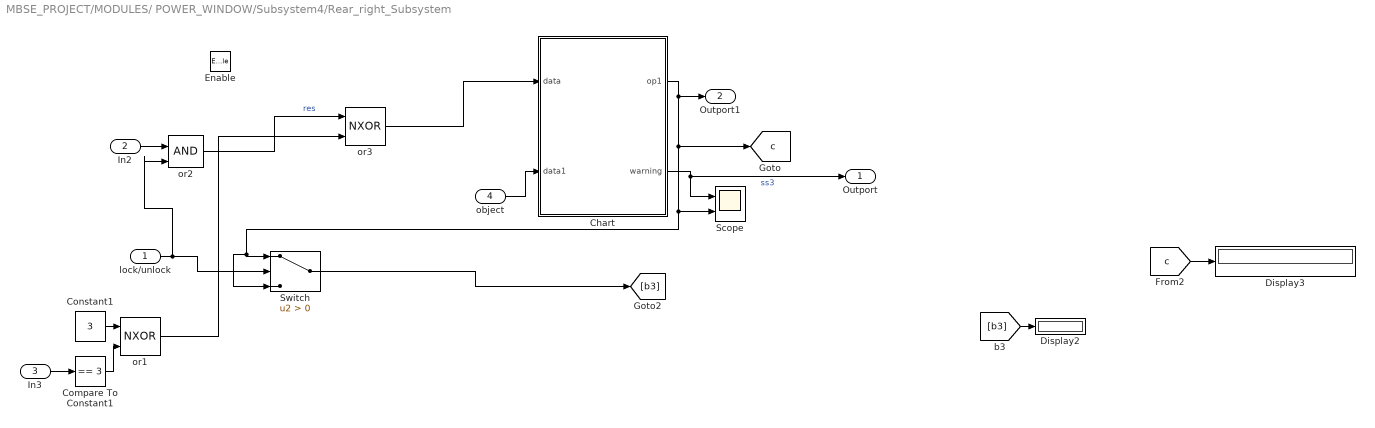
== system MBSE_PROJECT/MODULES/	POWER_WINDOW/Subsystem4/Rear_right_Subsystem ==
  lock/unlock : Inport
  In2 : Inport  Port=2
  In3 : Inport  Port=3
  object : Inport  Port=4
  Enable : EnablePort
  Chart : Stateflow chart  TreatAsAtomicUnit=on
  Compare To Constant1 : simulink/Logic and Bit Operations/Compare To Constant  relop===  const=3  OutDataTypeStr=boolean
  Constant1 : Constant  Value=3
  Display2 : Display
  Display3 : Display
  Scope : Scope  NumInputPorts=2
  Switch : Switch  Criteria=u2 > Threshold
  or1 : Logic  Operator=NXOR  IconShape=distinctive  AllPortsSameDT=off  OutDataTypeStr=boolean
  or2 : Logic  IconShape=distinctive  AllPortsSameDT=off  OutDataTypeStr=boolean
  or3 : Logic  Operator=NXOR  IconShape=distinctive  AllPortsSameDT=off  OutDataTypeStr=boolean
  Outport : Outport
  Outport1 : Outport  Port=2
  tag scope: c=global
  wires:
  Constant1/1 -> or1/1
  [b3] -> Display2/1
  Compare To Constant1/1 -> or1/2
  Switch/1 -> [b3]
  lock/unlock/1 -> or2/2, Switch/2
  Chart/2(warning) -> Scope/1, Outport/1  "ss3"
  object/1 -> Chart/2(data1)
  or1/1 -> or3/2
  or2/1 -> or3/1  "res"
  or3/1 -> Chart/1(data)
  [c] -> Display3/1
  Chart/1(op1) -> Outport1/1, [c], Scope/2, Switch/3, Switch/1
  In2/1 -> or2/1
  In3/1 -> Compare To Constant1/1

== system MBSE_PROJECT/MODULES/	POWER_WINDOW/Subsystem4/driver_control_Subsystem ==
  In1 : Inport
  object : Inport  Port=2
  Enable : EnablePort
  Chart : Stateflow chart  TreatAsAtomicUnit=on
  Display4 : Display
  Scope : Scope  NumInputPorts=2
  Outport : Outport
  Outport1 : Outport  Port=2
  tag scope: d=global
  wires:
  Chart/2(warning) -> Outport/1, Scope/1  "ss4"
  object/1 -> Chart/2(data1)
  In1/1 -> Chart/1(data)
  [d] -> Display4/1
  Chart/1(op1) -> Outport1/1, [d], Scope/2

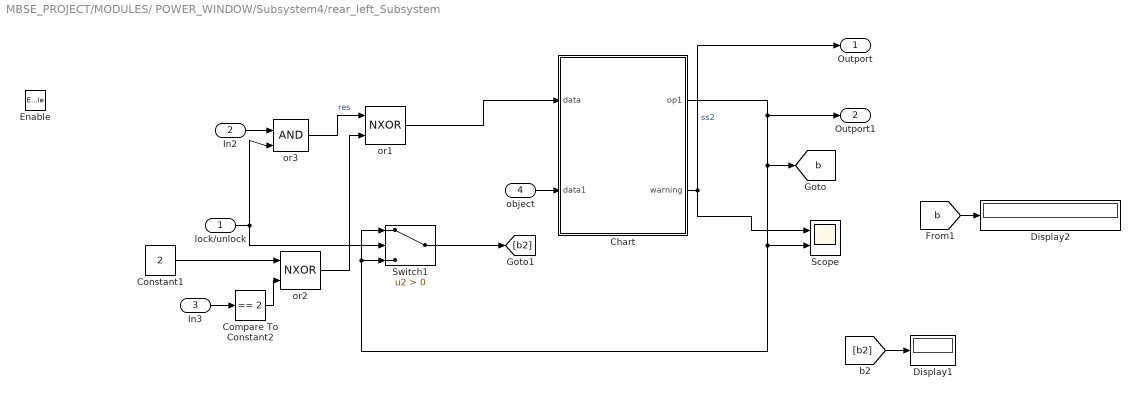
== system MBSE_PROJECT/MODULES/	POWER_WINDOW/Subsystem4/rear_left_Subsystem ==
  lock/unlock : Inport
  In2 : Inport  Port=2
  In3 : Inport  Port=3
  object : Inport  Port=4
  Enable : EnablePort
  Chart : Stateflow chart  TreatAsAtomicUnit=on
  Compare To Constant2 : simulink/Logic and Bit Operations/Compare To Constant  relop===  const=2  OutDataTypeStr=boolean
  Constant1 : Constant  Value=2
  Display1 : Display
  Display2 : Display
  Scope : Scope  NumInputPorts=2
  Switch1 : Switch  Criteria=u2 > Threshold
  or1 : Logic  Operator=NXOR  IconShape=distinctive  AllPortsSameDT=off  OutDataTypeStr=boolean
  or2 : Logic  Operator=NXOR  IconShape=distinctive  AllPortsSameDT=off  OutDataTypeStr=boolean
  or3 : Logic  IconShape=distinctive  AllPortsSameDT=off  OutDataTypeStr=boolean
  Outport : Outport
  Outport1 : Outport  Port=2
  tag scope: b=global
  wires:
  [b2] -> Display1/1
  Constant1/1 -> or2/1
  Compare To Constant2/1 -> or2/2
  Switch1/1 -> [b2]
  lock/unlock/1 -> Switch1/2, or3/2
  object/1 -> Chart/2(data1)
  Chart/2(warning) -> Outport/1, Scope/1  "ss2"
  or3/1 -> or1/1  "res"
  or2/1 -> or1/2
  or1/1 -> Chart/1(data)
  [b] -> Display2/1
  Chart/1(op1) -> Outport1/1, [b], Switch1/3, Switch1/1, Scope/2
  In2/1 -> or3/1
  In3/1 -> Compare To Constant2/1

== system MBSE_PROJECT/MODULES/AirBagSystem/FrontAirBagActivation/DriverFrontAirBagActive ==
  In1 : Inport
  Trigger : TriggerPort  VariantControl=(inherit)
  Constant : Constant
  Constant1 : Constant
  Constant2 : Constant
  Relational Operator : RelationalOperator  Operator===  OutDataTypeStr=boolean  RndMeth=Simplest
  Relational Operator1 : RelationalOperator  Operator===  OutDataTypeStr=boolean  RndMeth=Simplest
  Relational Operator2 : RelationalOperator  Operator===  OutDataTypeStr=boolean  RndMeth=Simplest
  tag scope: DriverAB=global, DriverDoor=global, FuelLock=global
  wires:
  In1/1 -> Relational Operator2/1, Relational Operator1/1, Relational Operator/1
  Constant/1 -> Relational Operator/2
  Constant1/1 -> Relational Operator1/2
  Constant2/1 -> Relational Operator2/2
  Relational Operator/1 -> [DriverAB]
  Relational Operator1/1 -> [DriverDoor]
  Relational Operator2/1 -> [FuelLock]

== system MBSE_PROJECT/MODULES/AirBagSystem/FrontAirBagActivation/LeftFrontAirBagActive ==
  In2 : Inport
  Trigger : TriggerPort  VariantControl=(inherit)
  Constant : Constant
  Constant1 : Constant
  Constant2 : Constant
  Relational Operator : RelationalOperator  Operator===  OutDataTypeStr=boolean  RndMeth=Simplest
  Relational Operator1 : RelationalOperator  Operator===  OutDataTypeStr=boolean  RndMeth=Simplest
  Relational Operator2 : RelationalOperator  Operator===  OutDataTypeStr=boolean  RndMeth=Simplest
  tag scope: FuelLock1=global, LeftFront=global, LeftFrontDoor=global
  wires:
  Constant1/1 -> Relational Operator1/2
  In2/1 -> Relational Operator2/1, Relational Operator1/1, Relational Operator/1
  Constant2/1 -> Relational Operator2/2
  Constant/1 -> Relational Operator/2
  Relational Operator/1 -> [LeftFront]
  Relational Operator1/1 -> [LeftFrontDoor]
  Relational Operator2/1 -> [FuelLock1]

== system MBSE_PROJECT/MODULES/AirBagSystem/FrontAirBagActivation/LeftRearAirBagActive ==
  In1 : Inport
  Trigger : TriggerPort  VariantControl=(inherit)
  Constant : Constant
  Constant1 : Constant
  Constant2 : Constant
  Relational Operator : RelationalOperator  Operator===  OutDataTypeStr=boolean  RndMeth=Simplest
  Relational Operator1 : RelationalOperator  Operator===  OutDataTypeStr=boolean  RndMeth=Simplest
  Relational Operator2 : RelationalOperator  Operator===  OutDataTypeStr=boolean  RndMeth=Simplest
  tag scope: FuelLock2=global, RearLeft=global, RearLeftDoor=global
  wires:
  Constant1/1 -> Relational Operator1/2
  In1/1 -> Relational Operator2/1, Relational Operator1/1, Relational Operator/1
  Constant2/1 -> Relational Operator2/2
  Constant/1 -> Relational Operator/2
  Relational Operator/1 -> [RearLeft]
  Relational Operator1/1 -> [RearLeftDoor]
  Relational Operator2/1 -> [FuelLock2]

== system MBSE_PROJECT/MODULES/AirBagSystem/FrontAirBagActivation/RightRearAirBagActive ==
  In2 : Inport
  Trigger : TriggerPort  VariantControl=(inherit)
  Constant : Constant
  Constant1 : Constant
  Constant2 : Constant
  Relational Operator : RelationalOperator  Operator===  OutDataTypeStr=boolean  RndMeth=Simplest
  Relational Operator1 : RelationalOperator  Operator===  OutDataTypeStr=boolean  RndMeth=Simplest
  Relational Operator2 : RelationalOperator  Operator===  OutDataTypeStr=boolean  RndMeth=Simplest
  tag scope: FuelLock3=global, RearRight=global, RearRightDoor=global
  wires:
  Constant1/1 -> Relational Operator1/2
  In2/1 -> Relational Operator2/1, Relational Operator1/1, Relational Operator/1
  Constant2/1 -> Relational Operator2/2
  Constant/1 -> Relational Operator/2
  Relational Operator/1 -> [RearRight]
  Relational Operator1/1 -> [RearRightDoor]
  Relational Operator2/1 -> [FuelLock3]

== system MBSE_PROJECT/MODULES/AirBagSystem/SideAirBagActivation/DriverSideAirBagActive ==
  In1 : Inport
  Trigger : TriggerPort  VariantControl=(inherit)
  Constant : Constant
  Constant1 : Constant
  Constant2 : Constant
  Relational Operator : RelationalOperator  Operator===  OutDataTypeStr=boolean  RndMeth=Simplest
  Relational Operator1 : RelationalOperator  Operator===  OutDataTypeStr=boolean  RndMeth=Simplest
  Relational Operator2 : RelationalOperator  Operator===  OutDataTypeStr=boolean  RndMeth=Simplest
  tag scope: DriverABSide=global, DriverDoorSide=global, FuelLockSide=global
  wires:
  In1/1 -> Relational Operator2/1, Relational Operator1/1, Relational Operator/1
  Constant/1 -> Relational Operator/2
  Constant1/1 -> Relational Operator1/2
  Constant2/1 -> Relational Operator2/2
  Relational Operator/1 -> [DriverABSide]
  Relational Operator1/1 -> [DriverDoorSide]
  Relational Operator2/1 -> [FuelLockSide]

== system MBSE_PROJECT/MODULES/AirBagSystem/SideAirBagActivation/LeftFronrSeatAirBagActive ==
  In2 : Inport
  Trigger : TriggerPort  VariantControl=(inherit)
  Constant : Constant
  Constant1 : Constant
  Constant2 : Constant
  Relational Operator : RelationalOperator  Operator===  OutDataTypeStr=boolean  RndMeth=Simplest
  Relational Operator1 : RelationalOperator  Operator===  OutDataTypeStr=boolean  RndMeth=Simplest
  Relational Operator2 : RelationalOperator  Operator===  OutDataTypeStr=boolean  RndMeth=Simplest
  tag scope: FuelLockSide1=global, LeftFrontDoorSide=global, LeftFrontSide=global
  wires:
  Constant1/1 -> Relational Operator1/2
  In2/1 -> Relational Operator2/1, Relational Operator1/1, Relational Operator/1
  Constant2/1 -> Relational Operator2/2
  Constant/1 -> Relational Operator/2
  Relational Operator/1 -> [LeftFrontSide]
  Relational Operator1/1 -> [LeftFrontDoorSide]
  Relational Operator2/1 -> [FuelLockSide1]

== system MBSE_PROJECT/MODULES/AirBagSystem/SideAirBagActivation/LeftRearAirBagActive ==
  In1 : Inport
  Trigger : TriggerPort  VariantControl=(inherit)
  Constant : Constant
  Constant1 : Constant
  Constant2 : Constant
  Relational Operator : RelationalOperator  Operator===  OutDataTypeStr=boolean  RndMeth=Simplest
  Relational Operator1 : RelationalOperator  Operator===  OutDataTypeStr=boolean  RndMeth=Simplest
  Relational Operator2 : RelationalOperator  Operator===  OutDataTypeStr=boolean  RndMeth=Simplest
  tag scope: FuelLockSide2=global, RearLeftDoorSide=global, RearLeftSide=global
  wires:
  Constant1/1 -> Relational Operator1/2
  In1/1 -> Relational Operator2/1, Relational Operator1/1, Relational Operator/1
  Constant2/1 -> Relational Operator2/2
  Constant/1 -> Relational Operator/2
  Relational Operator1/1 -> [RearLeftDoorSide]
  Relational Operator2/1 -> [FuelLockSide2]
  Relational Operator/1 -> [RearLeftSide]

== system MBSE_PROJECT/MODULES/AirBagSystem/SideAirBagActivation/RightRearAirBagActive ==
  In2 : Inport
  Trigger : TriggerPort  VariantControl=(inherit)
  Constant : Constant
  Constant1 : Constant
  Constant2 : Constant
  Relational Operator : RelationalOperator  Operator===  OutDataTypeStr=boolean  RndMeth=Simplest
  Relational Operator1 : RelationalOperator  Operator===  OutDataTypeStr=boolean  RndMeth=Simplest
  Relational Operator2 : RelationalOperator  Operator===  OutDataTypeStr=boolean  RndMeth=Simplest
  tag scope: FuelLockSide3=global, RearRightDoorSide=global, RearRightSide=global
  wires:
  Constant1/1 -> Relational Operator1/2
  In2/1 -> Relational Operator2/1, Relational Operator1/1, Relational Operator/1
  Constant2/1 -> Relational Operator2/2
  Constant/1 -> Relational Operator/2
  Relational Operator/1 -> [RearRightSide]
  Relational Operator1/1 -> [RearRightDoorSide]
  Relational Operator2/1 -> [FuelLockSide3]

== system MBSE_PROJECT/MODULES/SeatRestraintSystem/PowerSeat/PowerSeat ==
  ConditionCheck2 : Inport
  ConditionCheck3 : Inport  Port=2
  RearAdjEnable : Inport  Port=3
  SeatAdjEnable : Inport  Port=4
  CushionAdjEnable : Inport  Port=5
  Enable : EnablePort
  Cushion : Subsystem
  Enable Adjustment mode2 : Switch  Criteria=u2 > Threshold
  Enable Adjustment mode3 : Switch  Criteria=u2 > Threshold
  Raise/LowerCushion : Constant  Value=73.895833
  Raise/LowerCushion1 : Constant  Value=73.895833
  Raise/LowerSeat : Constant  Value=60
  Rear : Subsystem
  Seat : Subsystem
  SliderForCushionAdjust : SliderBlock
  SliderForSeatAdjust : SliderBlock
  "adjustment : Cushion" : Display
  "adjustment : Seat" : Display
  wires:
  Raise/LowerCushion/1 -> Enable Adjustment mode2/1
  ConditionCheck2/1 -> Enable Adjustment mode2/2
  ConditionCheck3/1 -> Enable Adjustment mode3/2
  Raise/LowerSeat/1 -> Enable Adjustment mode3/1
  Enable Adjustment mode2/1 -> "adjustment : Cushion"/1
  Enable Adjustment mode3/1 -> "adjustment : Seat"/1
  RearAdjEnable/1 -> Rear/1(PreviousEnable)
  [ModeSelection] -> Cushion/1(In1), Seat/1(In1), Rear/2(ModeSelection)
  SeatAdjEnable/1 -> Seat/2(EnableCheck)
  CushionAdjEnable/1 -> Cushion/2(EnableCheck)

== system MBSE_PROJECT/MODULES/Subsystem2/Subsystem/Enabled Subsystem ==
  In1 : Inport
  Enable : EnablePort
  Outport : Outport
  wires:
  In1/1 -> Outport/1

== system MBSE_PROJECT/MODULES/Subsystem2/Subsystem1/Enabled Subsystem1 ==
  In1 : Inport
  Enable : EnablePort
  Outport : Outport
  wires:
  In1/1 -> Outport/1

== system MBSE_PROJECT/MODULES/Subsystem4/AutomaticDoorLock/If Action Subsystem ==
  In1 : Inport
  Action Port : ActionPort  ActionPortLabel=if(u1>=13)
  Out1 : Outport
  wires:
  In1/1 -> Out1/1

== system MBSE_PROJECT/MODULES/Subsystem4/AutomaticDoorLock/If Action Subsystem1 ==
  In1 : Inport
  Action Port : ActionPort  ActionPortLabel=elseif(u1<13)
  Out1 : Outport
  wires:
  In1/1 -> Out1/1

== system MBSE_PROJECT/MODULES/Tire Pressure Monitoring System/TP_Monitoring/indicateHigh1 ==
  Enable : EnablePort
  Constant : Constant  Value=0
  Out1 : Outport
  wires:
  Constant/1 -> Out1/1

== system MBSE_PROJECT/MODULES/Tire Pressure Monitoring System/TP_Monitoring/indicateHigh2 ==
  Enable : EnablePort
  Constant : Constant  Value=0
  Out1 : Outport
  wires:
  Constant/1 -> Out1/1

== system MBSE_PROJECT/MODULES/Tire Pressure Monitoring System/TP_Monitoring/indicateHigh3 ==
  Enable : EnablePort
  Constant : Constant  Value=0
  Out1 : Outport
  wires:
  Constant/1 -> Out1/1

== system MBSE_PROJECT/MODULES/Tire Pressure Monitoring System/TP_Monitoring/indicateHigh4 ==
  Enable : EnablePort
  Constant : Constant  Value=0
  Out1 : Outport
  wires:
  Constant/1 -> Out1/1

== system MBSE_PROJECT/MODULES/Tire Pressure Monitoring System/TP_Monitoring/indicateLow1 ==
  Enable : EnablePort
  Constant : Constant
  Out1 : Outport
  wires:
  Constant/1 -> Out1/1

== system MBSE_PROJECT/MODULES/Tire Pressure Monitoring System/TP_Monitoring/indicateLow2 ==
  Enable : EnablePort
  Constant : Constant
  Out1 : Outport
  wires:
  Constant/1 -> Out1/1

== system MBSE_PROJECT/MODULES/Tire Pressure Monitoring System/TP_Monitoring/indicateLow3 ==
  Enable : EnablePort
  Constant : Constant
  Out1 : Outport
  wires:
  Constant/1 -> Out1/1

== system MBSE_PROJECT/MODULES/Tire Pressure Monitoring System/TP_Monitoring/indicateLow4 ==
  Enable : EnablePort
  Constant : Constant
  Out1 : Outport
  wires:
  Constant/1 -> Out1/1

== system MBSE_PROJECT/MODULES/SeatRestraintSystem/PowerSeat/PowerSeat/Cushion ==
  In1 : Inport
  EnableCheck : Inport  Port=2
  AND2 : Logic  IconShape=distinctive  AllPortsSameDT=off  OutDataTypeStr=boolean
  Constant2 : Constant
  CushionAdjustmentLogic : Subsystem  TreatAsAtomicUnit=on
  Relational Operator2 : RelationalOperator  Operator===  OutDataTypeStr=boolean  RndMeth=Simplest
  Relational Operator5 : RelationalOperator  Operator===  OutDataTypeStr=boolean  RndMeth=Simplest
  wires:
  Relational Operator5/1 -> CushionAdjustmentLogic/Enable, CushionAdjustmentLogic/1(EnableCheck)
  Relational Operator2/1 -> AND2/1
  AND2/1 -> Relational Operator5/1
  In1/1 -> Relational Operator2/1
  [CushionAdjustMode] -> Relational Operator2/2
  EnableCheck/1 -> AND2/2
  Constant2/1 -> Relational Operator5/2

== system MBSE_PROJECT/MODULES/SeatRestraintSystem/PowerSeat/PowerSeat/Rear ==
  PreviousEnable : Inport
  ModeSelection : Inport  Port=2
  AND : Logic  IconShape=distinctive  AllPortsSameDT=off  OutDataTypeStr=boolean
  Constant : Constant
  RearAdjustmentLogic : Subsystem  TreatAsAtomicUnit=on
  Relational Operator : RelationalOperator  Operator===  OutDataTypeStr=boolean  RndMeth=Simplest
  Relational Operator1 : RelationalOperator  Operator===  OutDataTypeStr=boolean  RndMeth=Simplest
  wires:
  [RearAdjustMode] -> Relational Operator/1
  PreviousEnable/1 -> AND/2
  Constant/1 -> Relational Operator1/2
  Relational Operator1/1 -> RearAdjustmentLogic/Enable, RearAdjustmentLogic/1(PreviousEnable)
  ModeSelection/1 -> Relational Operator/2
  AND/1 -> Relational Operator1/1
  Relational Operator/1 -> AND/1

== system MBSE_PROJECT/MODULES/SeatRestraintSystem/PowerSeat/PowerSeat/Seat ==
  In1 : Inport
  EnableCheck : Inport  Port=2
  AND1 : Logic  IconShape=distinctive  AllPortsSameDT=off  OutDataTypeStr=boolean
  Constant1 : Constant
  Relational Operator3 : RelationalOperator  Operator===  OutDataTypeStr=boolean  RndMeth=Simplest
  Relational Operator4 : RelationalOperator  Operator===  OutDataTypeStr=boolean  RndMeth=Simplest
  SeatAdjustmentLogic : Subsystem  TreatAsAtomicUnit=on
  wires:
  Constant1/1 -> Relational Operator4/2
  Relational Operator4/1 -> SeatAdjustmentLogic/1(EnableCheck), SeatAdjustmentLogic/Enable
  Relational Operator3/1 -> AND1/1
  AND1/1 -> Relational Operator4/1
  [SeatAdjustMode] -> Relational Operator3/2
  EnableCheck/1 -> AND1/2
  In1/1 -> Relational Operator3/1

== system MBSE_PROJECT/MODULES/SeatRestraintSystem/PowerSeat/PowerSeat/Cushion/CushionAdjustmentLogic ==
  EnableCheck : Inport
  Enable : EnablePort
  Compare To Constant : simulink/Logic and Bit Operations/Compare To Constant  relop=>  const=0  OutDataTypeStr=boolean
  CushionAdjust1 : LampBlock
  Switch : Switch  Criteria=u2 > Threshold
  tag scope: CushionAngle=global
  wires:
  EnableCheck/1 -> Switch/2
  [CushionAdjust] -> Switch/1
  Switch/1 -> Compare To Constant/1
  Compare To Constant/1 -> [CushionAngle]

== system MBSE_PROJECT/MODULES/SeatRestraintSystem/PowerSeat/PowerSeat/Rear/RearAdjustmentLogic ==
  PreviousEnable : Inport
  Enable : EnablePort
  Adjusted : simulink/Logic and Bit Operations/Compare To Constant  relop=>  const=0  OutDataTypeStr=boolean
  Switch : Switch  Criteria=u2 > Threshold
  tag scope: RearAngle=global
  wires:
  PreviousEnable/1 -> Switch/2
  [RearSide] -> Switch/1
  Switch/1 -> Adjusted/1
  Adjusted/1 -> [RearAngle]

== system MBSE_PROJECT/MODULES/SeatRestraintSystem/PowerSeat/PowerSeat/Seat/SeatAdjustmentLogic ==
  EnableCheck : Inport
  Enable : EnablePort
  SeatAdjustment : simulink/Logic and Bit Operations/Compare To Constant  relop=>  const=0  OutDataTypeStr=boolean
  Switch : Switch  Criteria=u2 > Threshold
  tag scope: SeatAngle=global
  wires:
  EnableCheck/1 -> Switch/2
  [SeatAdjust] -> Switch/1
  Switch/1 -> SeatAdjustment/1
  SeatAdjustment/1 -> [SeatAngle]

== stateflow chart MBSE_PROJECT/MODULES/	POWER_WINDOW/Subsystem4/Front_left_subsystem/decision_Box ==
  state Normal
    state Start
      entry:
      op1 = 25;
    state second
      entry:
      op1 = 100;
    state PrepareToStop
      entry:
      op1 = 75;
    state Go
      % Green light
      entry:
      op1 = 50;
    (default) -> Start
    Start -> (junction 9)
    (junction 9) -> (junction 6) : after(1,sec)
    PrepareToStop -> second : after(1,sec)
    (junction 6) -> Go
    Go -> PrepareToStop : after(1,sec)
  state Fault
    entry:
    op1 =0;
    state BlinkOn
      % Red light
      entry:
      warning = 1;
    (default) -> BlinkOn
  state block_start
    entry:
  state Normal2
    state state5
      entry:
      op1=0
    state Start1
      entry:
      op1=op1;
    state two
      entry:
      op1 = 0;
    state four3
      entry:
      op1 = 0;
    state three
      entry:
      op1 = 25;
    state three1
      entry:
      op1 = 0;
    state five2
      entry:
      op1=0;
    state five
      entry:
      op1=50;
    state five1
      entry:
      op1=25;
    state four2
      entry:
      op1 = 25;
    state four
      entry:
      op1 = 75;
    state four1
      entry:
      op1 = 50;
    Start1 -> state5 [order 4] : [op1==0]
    (default) -> Start1
    Start1 -> (junction 143) [order 2] : after(1,sec)[op1==25]
    (junction 143) -> four3
    Start1 -> (junction 89) [order 3]
    Start1 -> (junction 103) [order 5]
    Start1 -> (junction 48) [order 1]
    (junction 103) -> (junction 104) : after(1,sec)[op1==50]
    (junction 48) -> (junction 49) : after(1,sec)[op1==100]
    (junction 89) -> (junction 90) : after(1,sec)[op1==75]
    three -> two : after(1,sec)[op1==25]
    (junction 104) -> four2
    (junction 49) -> four
    five -> three : after(1,sec)[op1==50]
    (junction 90) -> four1
    five1 -> three1 : after(1,sec)[op1==25]
    four2 -> five2 : after(1,sec)[op1==25]
    four -> five : after(1,sec)[op1==75]
    four1 -> five1 : after(1,sec)[op1==50]
  (default) -> block_start
  block_start -> Normal2 [order 2] : [data == 0]
  Normal -> Fault [order 1] : [data1 == 1]
  block_start -> Normal [order 1] : [data ==1 ]
  Normal2 -> block_start [order 1] : [data ==1]
  Normal -> block_start [order 2] : [data == 0]
  Fault -> Normal [order 1] : [data1 == 0]
  Fault -> Normal2 [order 2] : [data1 ==0]
  Normal2 -> Fault [order 2] : [data1==1]
  data: data input; data1 input; op1 output =0; warning output
